simulink subsystem "magnetometer_sensor"  (R2023b)
settings: Solver=VariableStepAuto  StartTime=0.0  StopTime=10.0  RelTol=1e-3
undefined symbols (not defined in the file): sensor_data
settings Model: Creator=pierb  LastModifiedBy=pierb

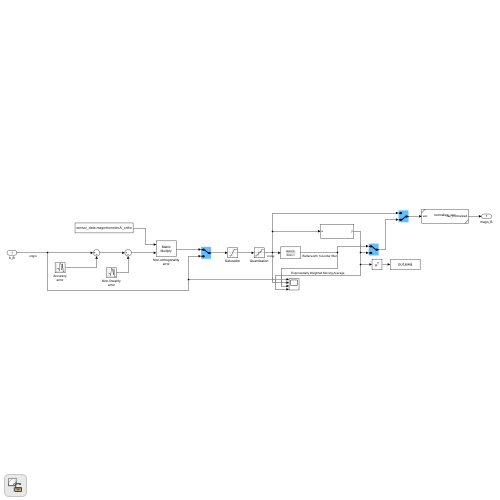
[thumbnail: Simulink's stored preview of the top-level diagram]
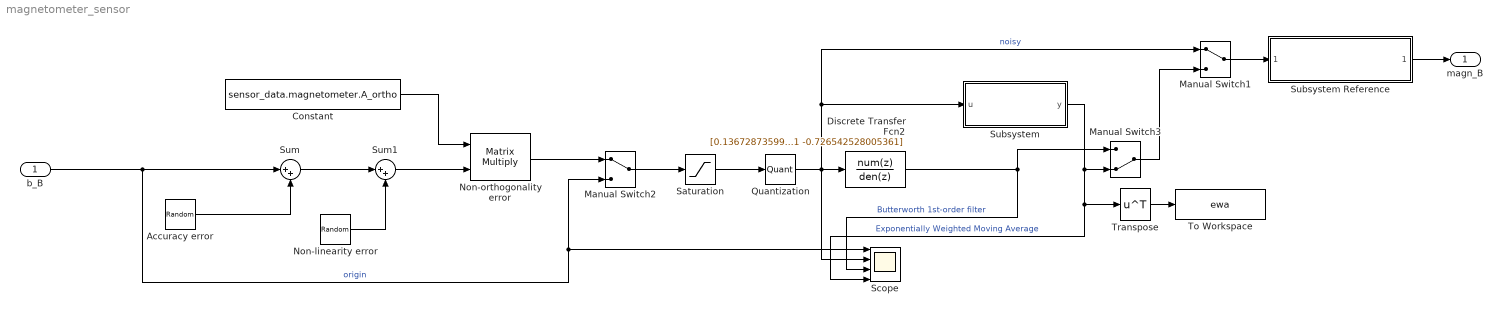
== system magnetometer_sensor ==
  b_B : Inport
  Accuracy error : RandomNumber  Variance=(sensor_data.magnetometer.acc/100*2*sensor_data.magnetometer.FSS)^2  Seed=[25 50 100]  SampleTime=1/sensor_data.magnetometer.freq
  Constant : Constant  Value=sensor_data.magnetometer.A_ortho
  Discrete Transfer Fcn2 : DiscreteTransferFcn  Numerator=[0.136728735997320 0.136728735997320]  Denominator=[1 -0.726542528005361]
  Manual Switch1 : ManualSwitch
  Manual Switch2 : ManualSwitch
  Manual Switch3 : ManualSwitch  CurrentSetting=0
  Non-linearity error : RandomNumber  Variance=(sensor_data.magnetometer.lin/100*2*sensor_data.magnetometer.FSS)^2  Seed=[200 400 800]  SampleTime=1/sensor_data.magnetometer.freq
  Non-orthogonality error : Product  Multiplication=Matrix(*)
  Quantization : Quantizer  QuantizationInterval=sensor_data.magnetometer.T_quant
  Saturation : Saturate  UpperLimit=sensor_data.magnetometer.FSS  LowerLimit=-sensor_data.magnetometer.FSS
  Scope : Scope  NumInputPorts=4
  Subsystem : Subsystem
  Subsystem Reference : Subsystem  ReferencedSubsystem=normalize_vec
  Sum : Sum  Inputs=|++
  Sum1 : Sum  Inputs=|++
  To Workspace : ToWorkspace  VariableName=ewa  SampleTime=-1
      settings: Save2DSignal=2-D array (concatenate along first dimension)
  Transpose : Math  Operator=transpose
  magn_B : Outport
  wires:
  Saturation/1 -> Quantization/1
  Sum/1 -> Sum1/1
  Accuracy error/1 -> Sum/2
  Non-linearity error/1 -> Sum1/2
  Sum1/1 -> Non-orthogonality error/2
  Constant/1 -> Non-orthogonality error/1
  Quantization/1 -> Discrete Transfer Fcn2/1, Subsystem/1(u), Manual Switch1/1, Scope/2  "noisy"
  b_B/1 -> Manual Switch2/2, Scope/1, Sum/1  "origin"
  Discrete Transfer Fcn2/1 -> Scope/3, Manual Switch3/1  "Butterworth 1st-order filter"
  Subsystem/1(y) -> Scope/4, Transpose/1, Manual Switch3/2  "Exponentially Weighted Moving Average"
  Transpose/1 -> To Workspace/1
  Manual Switch3/1 -> Manual Switch1/2
  Manual Switch1/1 -> Subsystem Reference/1
  Non-orthogonality error/1 -> Manual Switch2/1
  Manual Switch2/1 -> Saturation/1
  Subsystem Reference/1 -> magn_B/1

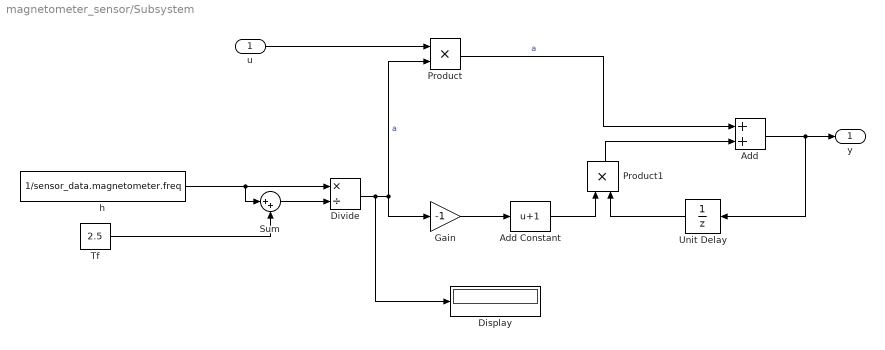
== system magnetometer_sensor/Subsystem ==
  u : Inport
  Add : Sum
  Add Constant : Bias  Bias=1  SaturateOnIntegerOverflow=off
  Display : Display
  Divide : Product  Inputs=*/
  Gain : Gain  Gain=-1
  Product : Product  Inputs=**
  Product1 : Product
  Sum : Sum  Inputs=|++
  Tf : Constant  Value=2.5
  Unit Delay : UnitDelay  SampleTime=-1  HasFrameUpgradeWarning=on
  h : Constant  Value=1/sensor_data.magnetometer.freq
  y : Outport
  wires:
  Product1/1 -> Add/2
  Unit Delay/1 -> Product1/2
  Add Constant/1 -> Product1/1
  Gain/1 -> Add Constant/1
  Product/1 -> Add/1  "a"
  u/1 -> Product/1
  Divide/1 -> Gain/1, Product/2, Display/1  "a"
  Tf/1 -> Sum/2
  Sum/1 -> Divide/2
  h/1 -> Divide/1, Sum/1
  Add/1 -> y/1, Unit Delay/1
